simulink model "mod2_SilveSteensgaard_inc"  (Simulink 7.9)
settings: Solver=ode45  StartTime=0.0  StopTime=simu.trantime  RelTol=1e-6
undefined symbols (not defined in the file): dc, DiscIntNeverNeededParam, Fs, mod, OSR, sinamp, sinfreq
libraries: simulink_extras x2, dsparch4 x1, simulink x1, dspsrcs4 x1
settings Model: Creator=Isacco Arnaldi  LastModifiedBy=Arnaldi Isacco
settings SolverCC: ZcThreshold=1e-6  ZeroCrossAlgorithm=Adaptive  AutoInsertRateTranBlk=on
settings DataIOCC: MaxDataPoints=50000  SaveOutput=off  SignalLogging=off  DSMLogging=off  SaveTime=off
settings OptimizationCC: InlineParams=on
settings DebuggingCC: StrictBusMsg=Warning
settings CodeAppCC: CustomSymbolStrType=$N$R$M_T
settings GRTTargetCC: CombineOutputUpdateFcns=off  GRTInterface=on

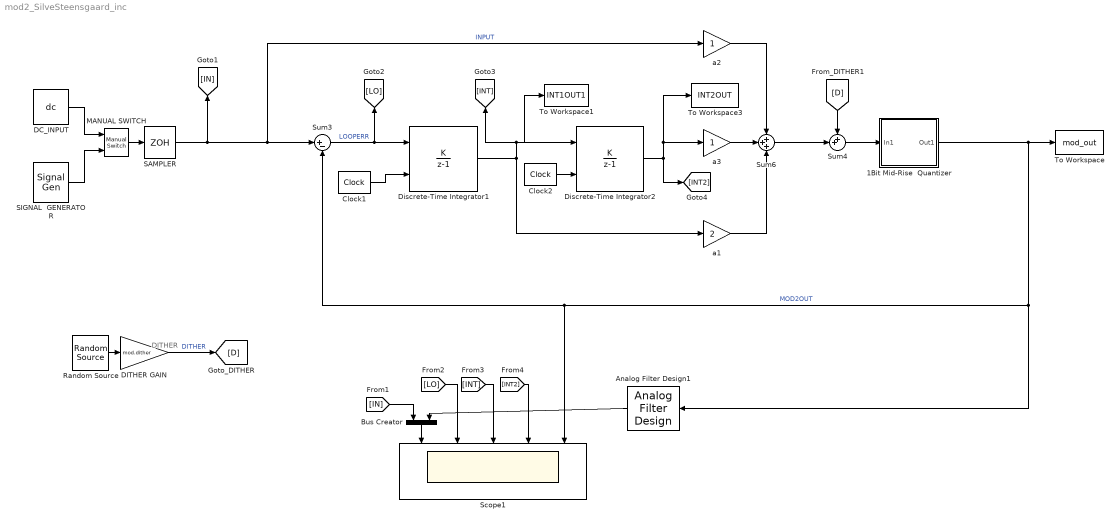
== system mod2_SilveSteensgaard_inc ==
  note: DITHER
  1Bit Mid-Rise  Quantizer : Subsystem
  Analog Filter Design1 : dsparch4/Analog Filter Design  method=Butterworth  filttype=Lowpass  N=8  Wlo=pi*(Fs/OSR)  Whi=80  Rp=2  Rs=40
  Bus Creator : BusCreator  Inputs=2
  Clock1 : simulink_extras/Flip Flops/Clock  period=1/(Fs/OSR)
  Clock2 : simulink_extras/Flip Flops/Clock  period=1/(Fs/OSR)
  DC_INPUT : Constant  Value=dc  OutDataTypeStr=double  SampleTime=1/(Fs/OSR)
  DITHER GAIN : Gain  Gain=mod.dither  SampleTime=1/Fs
  Discrete-Time Integrator1 : DiscreteIntegrator  IntegratorMethod=Accumulation: Forward Euler  ExternalReset=falling  SampleTime=1/Fs  LimitOutput=on  ICPrevOutput=DiscIntNeverNeededParam  ICPrevScaledInput=DiscIntNeverNeededParam
  Discrete-Time Integrator2 : DiscreteIntegrator  IntegratorMethod=Accumulation: Forward Euler  ExternalReset=rising  SampleTime=1/Fs  LimitOutput=on  ICPrevOutput=DiscIntNeverNeededParam  ICPrevScaledInput=DiscIntNeverNeededParam
  MANUAL SWITCH : simulink/Signal Routing/Manual Switch  sw=0  action=0  varsize=off
      settings: AttributesFormatString=Double click to\nselect the desired\ninput
  Random Source : dspsrcs4/Random Source  SrcType=Uniform  NormMethod=Ziggurat  CltLength=12  MinVal=-1  MaxVal=1  MeanVal=0  VarVal=1  RepMode=Not repeatable  rawSeed=1  IsInherit=off  SampMode=Discrete  SampTime=1/Fs  SampFrame=1  DataType=Double  OutComplex=Real
  SAMPLER : ZeroOrderHold  SampleTime=1/(Fs/OSR)
  SIGNAL  GENERATOR : SignalGenerator  Amplitude=sinamp  Frequency=sinfreq
  Scope1 : Scope  NumInputPorts=5
      settings: TimeRange=2.089895171320487e-05  YMin=-1.1~-0.6~-0.6~-0.3~-5  YMax=1.1~1.6~1.6~0.1~5
  Sum3 : Sum  Inputs=|+-  SampleTime=1/Fs
      settings: AttributesFormatString=Modulator Input\nLoop Error (input - fbk)
  Sum4 : Sum  Inputs=++|  SampleTime=1/Fs
  Sum6 : Sum  Inputs=+++  SampleTime=1/Fs
  To Workspace : ToWorkspace  VariableName=mod_out  SampleTime=-1
      settings: AttributesFormatString=Export output to\nworkspace for\npost-processing
  To Workspace1 : ToWorkspace  VariableName=INT1OUT1  SampleTime=-1
  To Workspace3 : ToWorkspace  VariableName=INT2OUT  SampleTime=-1
  a1 : Gain  Gain=2  SampleTime=1/Fs
  a2 : Gain  SampleTime=1/Fs
  a3 : Gain
  wires:
  Random Source/1 -> DITHER GAIN/1
  DITHER GAIN/1 -> [D]  "DITHER"
  DC_INPUT/1 -> MANUAL SWITCH/1
  SIGNAL  GENERATOR/1 -> MANUAL SWITCH/2
  MANUAL SWITCH/1 -> SAMPLER/1
  SAMPLER/1 -> [IN], Sum3/1, a2/1  "INPUT"
  [IN] -> Bus Creator/1
  Bus Creator/1 -> Scope1/1
  Analog Filter Design1/1 -> Bus Creator/2
  [LO] -> Scope1/2
  [INT] -> Scope1/3
  Sum3/1 -> Discrete-Time Integrator1/1, [LO]  "LOOPERR"
  Sum4/1 -> 1Bit Mid-Rise  Quantizer/1(In1)
  [D] -> Sum4/1
  1Bit Mid-Rise  Quantizer/1(Out1) -> To Workspace/1, Analog Filter Design1/1, Sum3/2, Scope1/5  "MOD2OUT"
  Sum6/1 -> Sum4/2
  a1/1 -> Sum6/3
  a2/1 -> Sum6/1
  a3/1 -> Sum6/2
  Clock1/1 -> Discrete-Time Integrator1/2
  Clock2/1 -> Discrete-Time Integrator2/2
  Discrete-Time Integrator1/1 -> Discrete-Time Integrator2/1, To Workspace1/1, [INT], a1/1
  Discrete-Time Integrator2/1 -> a3/1, To Workspace3/1, [INT2]
  [INT2] -> Scope1/4

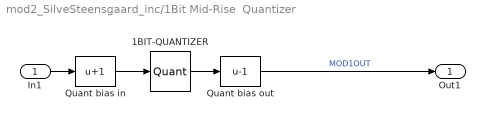
== system mod2_SilveSteensgaard_inc/1Bit Mid-Rise  Quantizer ==
  In1 : Inport
  1BIT-QUANTIZER : Quantizer  QuantizationInterval=2  SampleTime=1/Fs
      settings: AttributesFormatString=step = 2
  Quant bias in : Bias  Bias=1
      settings: AttributesFormatString=Need offset to give\nMID-RISE quantiser
  Quant bias out : Bias  Bias=-1
      settings: AttributesFormatString=Shift outputs to\n..., -2, 1, 1, ...
  Out1 : Outport
  wires:
  Quant bias out/1 -> Out1/1  "MOD1OUT"
  Quant bias in/1 -> 1BIT-QUANTIZER/1
  1BIT-QUANTIZER/1 -> Quant bias out/1
  In1/1 -> Quant bias in/1
